simulink model "Day1"  (R2017b)
settings: Solver=VariableStepAuto  StartTime=0.0  StopTime=10.0  MaxStep=1  RelTol=1e-3
undefined symbols (not defined in the file or in its folder): x1, x2, y1, y2
settings Model: Creator=Mahe  LastModifiedBy=Mahe

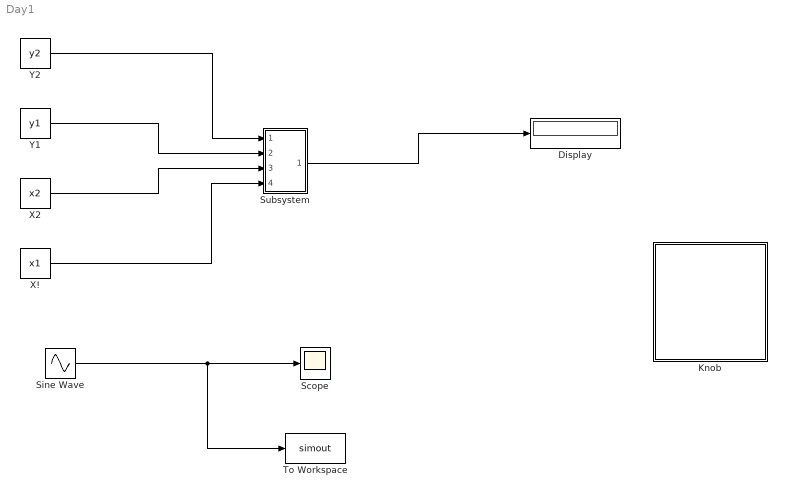
== system Day1 ==
  Display : Display
  Knob : Subsystem  DialogController=hmiCreateDDGDialog  IsWebBlock=on  mask(MWDashboardBlock){webBlockId=de870d72-3489-41a6-9e01-f9b40f700434, webBlockType=continuousknob, ShowInLibBrowser=on, ShowInitialText=on, HMISrcModelName=Day1}
      mask prompts: webBlockId "WebBlock Id"; webBlockType "WebBlock Type"; HMISrcModelName "Source Model"
      mask help: SimulinkHMI:dialogs:ContinuousKnobDialogDesc
      mask Help: helpview([docroot '/mapfiles/simulink.map'], 'hmi_knob')
      mask Display:
      | if strcmp(get_param(bdroot(gcb),'BlockDiagramType'), 'library')
      |     image([(matlabroot) '/toolbox/simulink/hmi/icons/ContinuousKnob.png']);
      | end
  Scope : Scope
  Sine Wave : Sin  SampleTime=0
  Subsystem : Subsystem
  To Workspace : ToWorkspace  VariableName=simout  SampleTime=-1
  X! : Constant  Value=x1
  X2 : Constant  Value=x2
  Y1 : Constant  Value=y1
  Y2 : Constant  Value=y2
  wires:
  Y2/1 -> Subsystem/1(In1)
  Y1/1 -> Subsystem/2(In2)
  X2/1 -> Subsystem/3(In3)
  X!/1 -> Subsystem/4(In4)
  Subsystem/1(Out1) -> Display/1
  Sine Wave/1 -> To Workspace/1, Scope/1

== system Day1/Knob ==

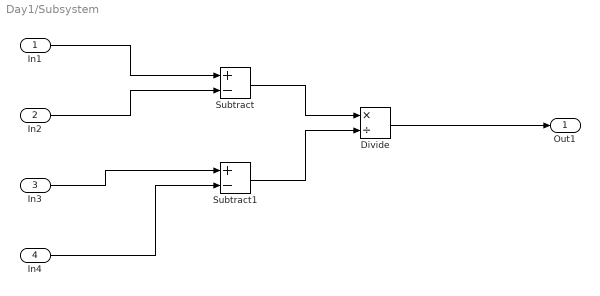
== system Day1/Subsystem ==
  In1 : Inport
  In2 : Inport  Port=2
  In3 : Inport  Port=3
  In4 : Inport  Port=4
  Divide : Product  Inputs=*/
  Subtract : Sum  Inputs=+-
  Subtract1 : Sum  Inputs=+-
  Out1 : Outport
  wires:
  Subtract1/1 -> Divide/2
  In1/1 -> Subtract/1
  Divide/1 -> Out1/1
  Subtract/1 -> Divide/1
  In3/1 -> Subtract1/1
  In4/1 -> Subtract1/2
  In2/1 -> Subtract/2
